simulink model "ex_separee_b"  (R2019a)
settings: Solver=VariableStepAuto  StartTime=0.0  StopTime=10.0  RelTol=1e-3
values from neighbouring files (symbols this model uses):
  Tl = 2.493    [ex_separee.m]
  Va = 24    [ex_separee.m]
  Vf = 12    [ex_separee.m]
libraries: powerlib x4
settings Model: Creator=azizi  LastModifiedBy=azizi

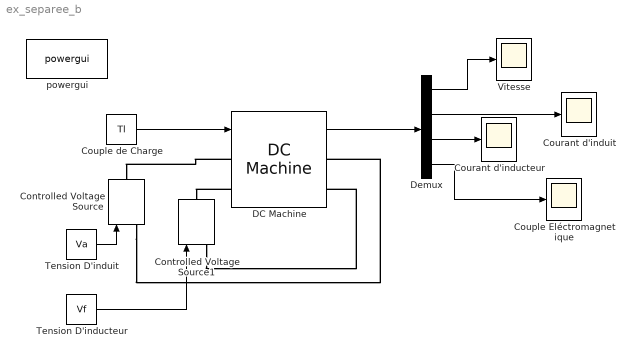
== system ex_separee_b ==
  Controlled Voltage Source : powerlib/Electrical Sources/Controlled Voltage Source  Initialize=on  Source_Type=AC  Amplitude=0  Phase=0  Frequency=0  Measurements=None
      settings: SourceProductName=Simscape Electrical
  Controlled Voltage Source1 : powerlib/Electrical Sources/Controlled Voltage Source  Initialize=on  Source_Type=AC  Amplitude=0  Phase=0  Frequency=0  Measurements=None
      settings: SourceProductName=Simscape Electrical
  Couple Eléctromagnetique : Scope
  Couple de Charge : Constant  Value=Tl
  Courant d'inducteur : Scope
  Courant d'induit : Scope
  DC Machine : powerlib/Machines/DC Machine  PresetModel=No  MechanicalLoad=Torque TL  FieldType=Wound  ShowDetailedParameters=on  MeasurementBus=off  RLa="[ 0.013  0.01]"  RLf="[ 1.43  0.167]"  Laf=0.004  MachineConstant=Torque constant (N.m/A)  Ke=1.8  Kt=1.8  J=0.21  Bm=1.074e-6  Tf=0  w0=1  Ifinit=1  TsPowergui=0  TsBlock=-1
      settings: SourceProductName=Simscape Electrical
  Demux : Demux
  Tension D'induit : Constant  Value=Va
  Tension D'inducteur : Constant  Value=Vf
  "Vitesse " : Scope
  powergui : powerlib/powergui  Priority=1  SimulationMode=Continuous  SampleTime=50e-6  frequency=60  Iterations=50  frequencyindice=0  Pbase=100e6  ErrMax=1e-4  UnitsV=kV  UnitsW=MW  buscounter=0  FunctionMessages=off  echomessages=off  EnableUseOfTLC=off  CurrentSourceSwitches=off  DisableSnubberDevices=off  DisableRonSwitches=off  DisableVfSwitches=off  DisplayEquations=off  AutomaticDiscreteSolvers=off  SolverType=Tustin/Backward Euler (TBE)  Interpol=off  ExternalGateDelay=off  methode=off  Ts=100  x0status=blocks  SPID=on  SwTol=0  HookPort=off  NonlinearTolerance=0  nMaxIteration=15  ContinueOnMaxIteration=off  RestoreLinks=warning  ResistiveCurrentMeasurement=off  Frange=[0:2:500]  Ylog=off  Xlog=on  ShowGrid=off  save=off  variable=ZData  structure=0  ZoomFFT=off  StartTime=0.0  cycles=1  DisplayStyle=1  fundamental=60  FreqAxis=off  MaxFrequency=1000  frequencyindicesteady=1  RmsSteady=1  display=off
      settings: SourceProductName=Simscape Electrical
  wires:
  Couple de Charge/1 -> DC Machine/1
  Tension D'induit/1 -> Controlled Voltage Source/1
  Tension D'inducteur/1 -> Controlled Voltage Source1/1
  DC Machine/1 -> Demux/1
  Demux/1 -> "Vitesse "/1
  Demux/2 -> Courant d'induit/1
  Demux/3 -> Courant d'inducteur/1
  Demux/4 -> Couple Eléctromagnetique/1
  connections:
  DC Machine/LConn1 -- Controlled Voltage Source/RConn1
  Controlled Voltage Source/LConn1 -- DC Machine/RConn1
  DC Machine/LConn2 -- Controlled Voltage Source1/RConn1
  Controlled Voltage Source1/LConn1 -- DC Machine/RConn2
